simulink model "mpc_model_dual_module_currentcontroller"  (R2019a)
settings: Solver=FixedStepAuto  StartTime=0.0  StopTime=Tfinal  RelTol=1e-3
values from neighbouring files (symbols this model uses):
  A = [-0.0285 -0.0014; -0.0371 -0.1476]    [model.m]
  DCLINK_Cap = 1000e-12    (= 1e-09)    [mpc_model_parameters.m]    (also in mpc_model_parameters_dual_module.m = 0.001)
  FluxPM = MeanInducedVoltagePeak/(2*pi*100)    [mpc_model_parameters.m]    (also in mpc_model_parameters_dual_module.m)
  Inertia = 1e-2    (= 0.01)    [mpc_model_parameters.m]    (also in mpc_model_parameters_dual_module.m)
  iqrated = Trated/(1.5*PolePairs*FluxPM)    [mpc_model_parameters.m]    (also in mpc_model_parameters_dual_module.m)
  Ki = 8    [mpc_model_parameters_dual_module.m]
  Kp = 0.8    [mpc_model_parameters_dual_module.m]
  Ls = 3.5e-3    (= 0.0035)    [MPC_id_iq.m]    (also in mpc_model_parameters.m = 0.00351; mpc_model_parameters_dual_module.m = 0.00343)
  M1_FaultTime = 0.25    [mpc_model_parameters_dual_module.m]
  M2_FaultTime = 20    [mpc_model_parameters_dual_module.m]
  MeanLd = (1/12)*(Module1Phase_A_Ld+Module1Phase_B_Ld+Module1Phase_C_Ld+     Module2Phase_A_Ld+Module2Phase_B_Ld+Module2Phase_C_Ld+     Module3Phase_A_Ld+Module3Phase_B_Ld+Module3Phase_C_Ld+     Module4Phase_A_Ld+Module4Phase_B_Ld+Module4Phase_C_Ld)    [mpc_model_parameters.m]    (also in mpc_model_parameters_dual_module.m)
  MeanLq = (1/12)*(Module1Phase_A_Lq+Module1Phase_B_Lq+Module1Phase_C_Lq+     Module2Phase_A_Lq+Module2Phase_B_Lq+Module2Phase_C_Lq+     Module3Phase_A_Lq+Module3Phase_B_Lq+Module3Phase_C_Lq+     Module4Phase_A_Lq+Module4Phase_B_Lq+Module4Phase_C_Lq)    [mpc_model_parameters.m]    (also in mpc_model_parameters_dual_module.m)
  PI_Frequency = 5000    [mpc_model_parameters_dual_module.m]
  PI_Sat = iqrated*2    [mpc_model_parameters_dual_module.m]
  PI_Ts = 1/PI_Frequency    (= 0.0002)    [mpc_model_parameters_dual_module.m]
  PolePairs = 10    [mpc_model_parameters.m]    (also in mpc_model_parameters_dual_module.m)
  RefModeSelection = 1    [mpc_model_parameters_dual_module.m]
  Rin = 1e-3    (= 0.001)    [mpc_model_parameters.m]    (also in mpc_model_parameters_dual_module.m)
  Rs = 0.531    [Loss_Distribution.m]    (also in MPC_id_iq.m; mpc_model_parameters.m = 0.321; mpc_model_parameters_dual_module.m = 0.539)
  Sampling_time = 1e-6    (= 1e-06)    [mpc_model_parameters.m]    (also in mpc_model_parameters_dual_module.m)
  SpeedRef1 = 50    [mpc_model_parameters.m]    (also in mpc_model_parameters_dual_module.m = 35)
  SpeedRef2 = 100    [mpc_model_parameters.m]    (also in mpc_model_parameters_dual_module.m = 35)
  SpeedRefUpdateTime = 0.25    [mpc_model_parameters.m]    (also in mpc_model_parameters_dual_module.m = 1.75)
  Tload1 = 5    [mpc_model_parameters.m]    (also in mpc_model_parameters_dual_module.m = 30)
  Tload2 = 10    [mpc_model_parameters.m]    (also in mpc_model_parameters_dual_module.m = 63.6619772368)
  TloadUpdateTime = 0.5    [mpc_model_parameters.m]    (also in mpc_model_parameters_dual_module.m)
  Vdc = 50    [mpc_model_parameters.m]    (also in mpc_model_parameters_dual_module.m = 40)
  Vin = Vdc + Rin*(Pout/Vdc)    (= 50.04)    [mpc_model_parameters.m]    (also in mpc_model_parameters_dual_module.m = 40.05)
  ViscousFriction = 1e-3    (= 0.001)    [mpc_model_parameters.m]    (also in mpc_model_parameters_dual_module.m)
undefined symbols (not defined in the file or in its folder): DiscIntNeverNeededParam, LoadResistance, VoltageConstant_omega
libraries: dspsigops x30, powerlib x27, dspswit3 x19, powerlib_meascontrol x11, fl_lib x5, simulink x4, nesl_utility x3, sdl_lib x1
(part 1 of 3)
settings Model: Creator=hakan  LastModifiedBy=hakan
settings SolverCC: ZeroCrossAlgorithm=Adaptive
settings DebuggingCC: IgnoredZcDiagnostic=none  UnconnectedInputMsg=none  UnconnectedOutputMsg=none  UnconnectedLineMsg=none

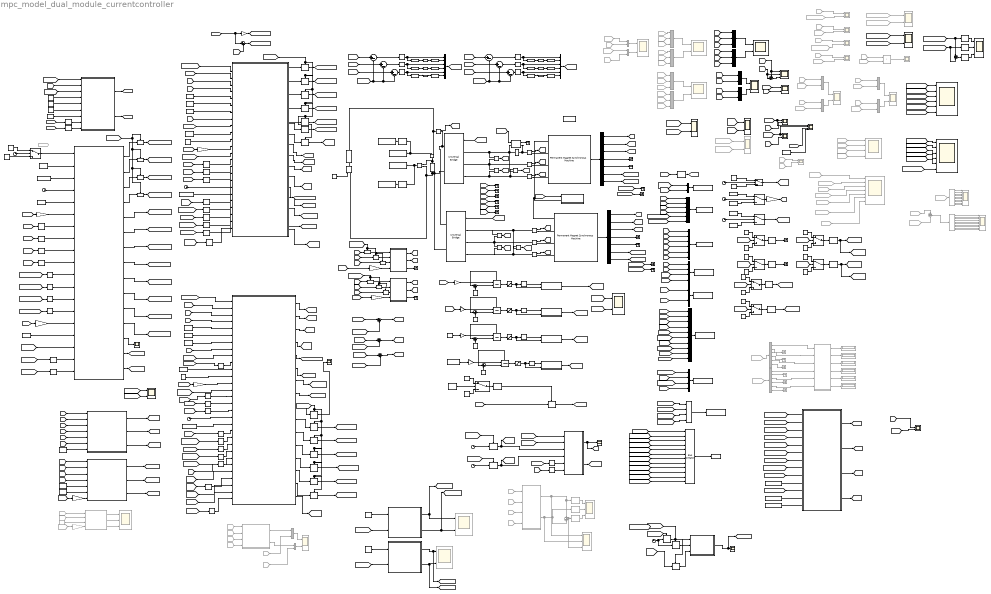
== system mpc_model_dual_module_currentcontroller ==
  note: M1_thetam & M2_thetam will be the but they are seperated anyway
  A_DCLINK_current : ToWorkspace  VariableName=M1_DCLINK_current  SaveFormat=Structure With Time  SampleTime=-1
  A_DCLINK_current_rms : ToWorkspace  VariableName=M1_DCLINK_current_rms  SaveFormat=Structure With Time  SampleTime=-1
  A_DCLINK_voltage : ToWorkspace  VariableName=M1_DCLINK_voltage  SaveFormat=Structure With Time  SampleTime=-1
  A_DCLINK_voltage_mean : ToWorkspace  VariableName=M1_DCLINK_voltage_mean  SaveFormat=Structure With Time  SampleTime=-1
  Bus Creator : BusCreator  Inputs=6
  Bus Creator1 : BusCreator  Inputs=6
  Bus Creator{3,10..12} (4 alike) : BusCreator  Inputs=2
  Bus Creator{13..14,17..20} (6 alike) : BusCreator  Commented=on  Inputs=2
  Bus Creator15 : BusCreator  Inputs=10
  Bus Creator16 : BusCreator  Inputs=4
  Bus Creator2 : BusCreator  Inputs=4
  Bus Creator21 : BusCreator  Inputs=4
  Bus Creator22 : BusCreator  Inputs=12
  Bus Creator{4..7} (4 alike) : BusCreator  Commented=on  Inputs=3
  Bus Creator8 : BusCreator  Inputs=3
  Bus Creator9 : BusCreator  Inputs=3
  Bus Selector : BusSelector  OutputSignals=Electromagnetic torque Te (N*m),Rotor speed wm (rad/s),Rotor angle thetam (rad),Stator current is_q (A),Stator current is_d (A),Stator voltage Vs_q (V),Stator voltage Vs_d (V)
  Bus Selector1 : BusSelector  OutputSignals=Electromagnetic torque Te (N*m),Rotor speed wm (rad/s),Rotor angle thetam (rad),Stator current is_q (A),Stator current is_d (A),Stator voltage Vs_q (V),Stator voltage Vs_d (V)
  Clock{,1..9} (10 alike) : Clock
  Compare To Zero{,1..3} (4 alike) : simulink/Logic and Bit Operations/Compare To Zero  relop===  OutDataTypeStr=boolean
  Constant : Constant  Value=Vin
  Constant{1..2,18,32} (4 alike) : Constant  Value=Rs
  Constant10 : Constant  Value=SpeedRef1
  Constant11 : Constant  Value=SpeedRef2
  Constant12 : Constant  Value=Tload2
  Constant13 : Constant  Value=M2_FaultTime
  Constant{5,14,26,31} (4 alike) : Constant  Value=Ls
  Constant{15,17,22,29,36,38..39,43,50,52} (10 alike) : Constant  Value=0
  Constant{16,23,27,30,37,44,49,51} (8 alike) : Constant
  Constant19 : Constant  Value=PolePairs
  Constant{4,6,20,34} (4 alike) : Constant  Value=FluxPM
  Constant21 : Constant  Value=Vdc
  Constant{7,24..25,41} (4 alike) : Constant  Value=1.02
  Constant28 : Constant  Value=M1_FaultTime
  Constant3 : Constant  Value=M1_FaultTime
  Constant33 : Constant  Value=PolePairs
  Constant35 : Constant  Value=Vdc
  Constant40 : Constant  Value=RefModeSelection
  Constant42 : Constant  Value=PI_Frequency
  Constant45 : Constant  Value=Ki
  Constant46 : Constant  Value=Kp
  Constant47 : Constant  Value=PI_Ts
  Constant48 : Constant  Value=PI_Sat
  Constant53 : Constant  Commented=on  Value=0
  Constant54 : Constant  Value=2*iqrated
  Constant55 : Constant  Value=5
  Constant56 : Constant  Value=15
  Constant8 : Constant  Value=Tload1
  Constant9 : Constant  Value=2000
  Controlled Voltage Source : powerlib/Electrical Sources/Controlled Voltage Source  Initialize=on  Source_Type=DC  Amplitude=0  Phase=0  Frequency=0  Measurements=None
      settings: SourceProductName=Simscape Electrical
  Current Measurement{,1..7} (8 alike) : powerlib/Measurements/Current Measurement  PhasorSimulation=off  OutputType=Complex  PSBequivalent=0
      settings: SourceProductName=Simscape Electrical
  DCLINK_Cap : powerlib/Elements/Series RLC Branch  LConnTagsString=__new0  RConnTagsString=__new0  BranchType=C  Resistance=1  Inductance=1e-3  SetiL0=off  InitialCurrent=0  Capacitance=DCLINK_Cap  Setx0=on  InitialVoltage=Vin  Measurements=None
      settings: SourceProductName=Simscape Electrical
  Data Type Conversion{1,3,5,12,14,16} (6 alike) : DataTypeConversion  OutDataTypeStr=boolean
  Data Type Conversion{2,4,6,13,15,17} (6 alike) : DataTypeConversion  OutDataTypeStr=double
  Delay{,1..21,23..29,32..33} (31 alike) : Delay  DelayLength=1
  Delay22 : Delay  DelayLength=1  InitialCondition=1
  Delay30 : Delay  DelayLength=1  InitialCondition=1
  Delay31 : Delay
  Demux : Demux  Commented=on  Outputs=10
  Demux1 : Demux  Commented=on  Outputs=10
  Demux2 : Demux  Commented=on  Outputs=6
  Demux3 : Demux  Commented=on  Outputs=6
  Discrete-Time Integrator{1..4} (4 alike) : DiscreteIntegrator  ExternalReset=falling  SampleTime=Sampling_time  UpperSaturationLimit=1  LowerSaturationLimit=0  ShowStatePort=on  ICPrevOutput=DiscIntNeverNeededParam  ICPrevScaledInput=DiscIntNeverNeededParam
  Display{1..6} (6 alike) : Display  Commented=on
  Edge Detector{1,3,5..9} (7 alike) : dspswit3/Edge Detector  InputProcessing=Columns as channels (frame based)
      settings: SourceProductName=DSP System Toolbox  SourceProductBaseCode=DS
  Error : Scope  Commented=on  NumInputPorts=10
  From10 : From  Commented=on  GotoTag=M1_Vbc
  From11 : From  Commented=on  GotoTag=M1_Vca
  From112 : From  Commented=on  GotoTag=PI_output
  From122 : From  Commented=on  GotoTag=M2_thetam
  From{126,172,246,250,262} (5 alike) : From  Commented=on  GotoTag=M2_ids
  From{49,127,171,244,248,260} (6 alike) : From  Commented=on  GotoTag=M1_ids
  From131 : From  Commented=on  GotoTag=M1_idref
  From137 : From  Commented=on  GotoTag=M1_cond_loss
  From138 : From  Commented=on  GotoTag=M1_core_loss
  From139 : From  Commented=on  GotoTag=M2_core_loss
  From140 : From  Commented=on  GotoTag=M2_cond_loss
  From141 : From  Commented=on  GotoTag=Total_cond_loss
  From142 : From  Commented=on  GotoTag=Total_core_loss
  From{143,166,242,311} (4 alike) : From  Commented=on  GotoTag=M1_iqref
  From144 : From  Commented=on  GotoTag=M2_iqref
  From{94,146,245,249,261} (5 alike) : From  Commented=on  GotoTag=M1_iqs
  From{148,247,251,263} (4 alike) : From  Commented=on  GotoTag=M2_iqs
  From156 : From  Commented=on  GotoTag=Total_loss
  From158 : From  Commented=on  GotoTag=Total_loss
  From159 : From  Commented=on  GotoTag=M2_loss
  From160 : From  Commented=on  GotoTag=M1_loss
  From161 : From  Commented=on  GotoTag=Mean_loss
  From164 : From  Commented=on  GotoTag=M1_opt
  From165 : From  Commented=on  GotoTag=M2_opt
  From167 : From  Commented=on  GotoTag=M2_iqref
  From170 : From  Commented=on  GotoTag=M2_idref
  From20 : From  Commented=on  GotoTag=M2_IqRipplePrediction
  From234 : From  Commented=on  GotoTag=M1_magneticloss
  From235 : From  Commented=on  GotoTag=M2_magneticloss
  From238 : From  Commented=on  GotoTag=M1_wmech
  From239 : From  Commented=on  GotoTag=M1_Te
  From240 : From  Commented=on  GotoTag=M2_idref
  From241 : From  Commented=on  GotoTag=M2_iqref
  From243 : From  Commented=on  GotoTag=M1_idref
  From252 : From  Commented=on  GotoTag=M1_Te
  From253 : From  Commented=on  GotoTag=M2_Te
  From309 : From  Commented=on  GotoTag=iq_2_store
  From310 : From  Commented=on  GotoTag=iq_2_store
  From32 : From  Commented=on  GotoTag=M1_va_1
  From33 : From  Commented=on  GotoTag=M1_vb_1
  From34 : From  Commented=on  GotoTag=M1_vc_1
  From42 : From  Commented=on  GotoTag=M1_mpcgate
  From58 : From  Commented=on  GotoTag=M2_Vbc
  From59 : From  Commented=on  GotoTag=M2_Vca
  From6 : From  Commented=on  GotoTag=M1_mpcgate
  From60 : From  Commented=on  GotoTag=M2_Vab
  From61 : From  Commented=on  GotoTag=M2_va_1
  From62 : From  Commented=on  GotoTag=M2_vb_1
  From63 : From  Commented=on  GotoTag=M2_vc_1
  From76 : From  Commented=on  GotoTag=M1_IqRipplePrediction
  From9 : From  Commented=on  GotoTag=M1_Vab
  Gain1 : Gain  Gain=2*pi/60
  Gain11 : Gain  Gain=0.5
  Gain{7..8,12,14} (4 alike) : Gain  Gain=2
  Gain{3..6,9,13,15} (7 alike) : Gain  Gain=PolePairs
  Gain2 : Gain  Commented=on  Gain=PolePairs
  Ideal Switch : powerlib/Power Electronics/Ideal Switch  Ron=0.001  Lon=0  IC=0  Rs=1e5  Cs=inf  Measurements=on
      settings: SourceProductName=Simscape Electrical
  Inverter1 : powerlib/Power Electronics/Universal Bridge  Arms=3  SnubberResistance=1e5  SnubberCapacitance=inf  Device=IGBT / Diodes  Ron=0.65e-3  Lon=0  ForwardVoltages="[  0  0  ]"  ForwardVoltage=0  GTOparameters=[ 10e-6 , 20e-6 ]  IGBTparameters=[ 1e-6 , 2e-6 ]  Measurements=All voltages and currents  Measurements_2=None  converterType=Rectifier
      settings: SourceProductName=Simscape Electrical
  Inverter2 : powerlib/Power Electronics/Universal Bridge  Arms=3  SnubberResistance=1e5  SnubberCapacitance=inf  Device=IGBT / Diodes  Ron=0.65e-3  Lon=0  ForwardVoltages="[  0  0  ]"  ForwardVoltage=0  GTOparameters=[ 10e-6 , 20e-6 ]  IGBTparameters=[ 1e-6 , 2e-6 ]  Measurements=All voltages and currents  Measurements_2=None  converterType=Rectifier
      settings: SourceProductName=Simscape Electrical
  Logical Operator{1..3,6..8} (6 alike) : Logic  Operator=NOT  AllPortsSameDT=off  OutDataTypeStr=boolean
  M1 Prediction : MATLAB Function  TreatAsAtomicUnit=on
  M2 Prediction : MATLAB Function  TreatAsAtomicUnit=on
  MATLAB Function : MATLAB Function  Commented=on  TreatAsAtomicUnit=on
  MATLAB Function1 : MATLAB Function  TreatAsAtomicUnit=on
  MATLAB Function10 : MATLAB Function  TreatAsAtomicUnit=on
  MATLAB Function11 : MATLAB Function  Commented=on  TreatAsAtomicUnit=on
  MATLAB Function12 : MATLAB Function  Commented=on  TreatAsAtomicUnit=on
  MATLAB Function13 : MATLAB Function  TreatAsAtomicUnit=on
  MATLAB Function14 : MATLAB Function  TreatAsAtomicUnit=on
  MATLAB Function15 : MATLAB Function  TreatAsAtomicUnit=on
  MATLAB Function2 : MATLAB Function  TreatAsAtomicUnit=on
  MATLAB Function3 : MATLAB Function  TreatAsAtomicUnit=on
  MATLAB Function4 : MATLAB Function  TreatAsAtomicUnit=on
  MATLAB Function5 : MATLAB Function  TreatAsAtomicUnit=on
  MATLAB Function6 : MATLAB Function  TreatAsAtomicUnit=on
  MATLAB Function7 : MATLAB Function  TreatAsAtomicUnit=on
  MATLAB Function8 : MATLAB Function  TreatAsAtomicUnit=on
  MATLAB Function9 : MATLAB Function  TreatAsAtomicUnit=on
  Mean : powerlib_meascontrol/Measurements/Mean  Freq=THD_mean_frequency  Vinit=0  Ts=Sampling_time
      settings: SourceProductName=Simscape Electrical
  Mean Switching Frequency : Subsystem  Commented=on
  Mean1 : powerlib_meascontrol/Measurements/Mean  Freq=1/0.2  Vinit=0  Ts=0
      settings: SourceProductName=Simscape Electrical
  Mean2 : powerlib_meascontrol/Measurements/Mean  Freq=5  Vinit=0  Ts=Sampling_time
      settings: SourceProductName=Simscape Electrical
  Mean3 : powerlib_meascontrol/Measurements/Mean  Freq=1/0.2  Vinit=0  Ts=0
      settings: SourceProductName=Simscape Electrical
  Mean4 : powerlib_meascontrol/Measurements/Mean  Freq=1/0.2  Vinit=0  Ts=0
      settings: SourceProductName=Simscape Electrical
  Mean5 : powerlib_meascontrol/Measurements/Mean  Commented=on  Freq=1/0.2  Vinit=0  Ts=0
      settings: SourceProductName=Simscape Electrical
  Mean6 : powerlib_meascontrol/Measurements/Mean  Commented=on  Freq=1/0.2  Vinit=0  Ts=0
      settings: SourceProductName=Simscape Electrical
  Mean7 : powerlib_meascontrol/Measurements/Mean  Commented=on  Freq=1/0.2  Vinit=0  Ts=0
      settings: SourceProductName=Simscape Electrical
  Mechanical Subsystem : Subsystem
  Multimeter : powerlib/Measurements/Multimeter  PhasorSimulation=off  OutputType=Complex  sel=27  L=32  Gain=1  yselected={'Isw1: Inverter1'};  PSBOutputType=1  PSBequivalent=0  AxesSetting=[0,0.1,-100,100]  Display=0  SavedBlockNames=-11
      settings: SourceProductName=Simscape Electrical
  Multimeter1 : powerlib/Measurements/Multimeter  PhasorSimulation=off  OutputType=Complex  sel=21  L=32  Gain=1  yselected={'Isw1: Inverter2'};  PSBOutputType=1  PSBequivalent=0  AxesSetting=[0,0.1,-100,100]  Display=0  SavedBlockNames=-11
      settings: SourceProductName=Simscape Electrical
  Mux : Mux  Commented=on  Inputs=2
  Mux1 : Mux  Inputs=6
  Mux2 : Mux  Commented=on  Inputs=2
  Mux4 : Mux  Inputs=6
  Permanent Magnet Synchronous Machine : powerlib/Machines/Permanent Magnet Synchronous Machine  NbPhases=3  FluxDistribution=Sinusoidal  RotorType=Round  MechanicalLoad=Mechanical rotational port  PresetModel=No  ShowDetailedParameters=on  MeasurementBus=off  Resistance=Rs  Inductance=8.5e-3  dqInductances=[MeanLd,MeanLq]  La=Ls  MachineConstant=Flux linkage established by magnets (V.s)  Flux=0.18074  VoltageCst=327.8261  TorqueCst=2.7111  Flat=120  Mechanical=[Inertia ViscousFriction PolePairs 0]  PolePairs=4  InitialConditions=[0,0, 0,0]  InitialConditions5ph=[0 0 0 0 0 0]  TsPowergui=0  TsBlock=-1  RefAngle=90 degrees behind phase A axis (modified Park)
  Permanent Magnet Synchronous Machine1 : powerlib/Machines/Permanent Magnet Synchronous Machine  NbPhases=3  FluxDistribution=Sinusoidal  RotorType=Round  MechanicalLoad=Mechanical rotational port  PresetModel=No  ShowDetailedParameters=on  MeasurementBus=off  Resistance=Rs  Inductance=8.5e-3  dqInductances=[MeanLd,MeanLq]  La=Ls  MachineConstant=Flux linkage established by magnets (V.s)  Flux=0.18074  VoltageCst=327.8261  TorqueCst=2.7111  Flat=120  Mechanical=[Inertia ViscousFriction PolePairs 0]  PolePairs=4  InitialConditions=[0,0, 0,0]  InitialConditions5ph=[0 0 0 0 0 0]  TsPowergui=0  TsBlock=-1  RefAngle=90 degrees behind phase A axis (modified Park)
  Product : Product  Commented=on
  RMS1 : powerlib_meascontrol/Measurements/RMS  TrueRMS=on  Freq=Load_Nominal_Freq  RMSInit=10  Ts=Sampling_time
      settings: SourceProductName=Simscape Electrical
  Relay{,1..5} (6 alike) : Relay
  Rin : powerlib/Elements/Series RLC Branch  LConnTagsString=__new0  RConnTagsString=__new0  BranchType=R  Resistance=Rin  Inductance=1e-3  SetiL0=off  InitialCurrent=0  Capacitance=1000e-6  Setx0=off  InitialVoltage=0  Measurements=None
      settings: SourceProductName=Simscape Electrical
  Sample and Hold{,1..29} (30 alike) : dspsigops/Sample and Hold  trig=Rising edge  initCond=0  latchinput=off
  Saturation{1..3,12} (4 alike) : Saturate  UpperLimit=1  LowerLimit=0
  Sawtooth Generator : powerlib_meascontrol/Pulse & Signal Generators/Sawtooth Generator  Freq=1000  Phase=180  Ts=0
      settings: SourceProductName=Simscape Electrical
  Scope : Scope  NumInputPorts=3
  Scope{1,5..6,8..10,12..13,22,30,35} (11 alike) : Scope  NumInputPorts=2
  Scope{2,4,7,11,17..19,21,24..28,37..38} (15 alike) : Scope  Commented=on  NumInputPorts=2
  Scope14 : Scope  Commented=on  NumInputPorts=3
  Scope{15,29,34,39} (4 alike) : Scope
  Scope16 : Scope  Commented=on  NumInputPorts=4
  Scope20 : Scope  NumInputPorts=4
  Scope23 : Scope  Commented=on
  Scope3 : Scope  Commented=on  NumInputPorts=7
  Scope31 : Scope  NumInputPorts=3
  Scope32 : Scope  Commented=on  NumInputPorts=3
  Scope33 : Scope  Commented=on  NumInputPorts=3
  Scope36 : Scope  NumInputPorts=6
  Scope40 : Scope  NumInputPorts=6
  Scope42 : Scope  Commented=on  NumInputPorts=10
  Series RLC Branch : powerlib/Elements/Series RLC Branch  LConnTagsString=__new0  RConnTagsString=__new0  BranchType=R  Resistance=5000  Inductance=1e-3  SetiL0=off  InitialCurrent=0  Capacitance=1e-6  Setx0=off  InitialVoltage=0  Measurements=None
      settings: SourceProductName=Simscape Electrical
  Sum : Sum  Inputs=|++
  Sum1 : Sum  Inputs=++|
  Sum{10..12,15} (4 alike) : Sum  Inputs=|-+
  Sum{2,4..6,8..9,13} (7 alike) : Sum  Inputs=|+-
  Sum14 : Sum
  Sum16 : Sum  Commented=on
  Sum18 : Sum  Commented=on  Inputs=+-
  Sum3 : Sum  Inputs=|++
  Sum7 : Sum  Inputs=|++
  Switch : Switch  Criteria=u2 > Threshold  Threshold=SpeedRefUpdateTime
  Switch1 : Switch  Criteria=u2 > Threshold  Threshold=TloadUpdateTime
  Switch11 : Switch  Criteria=u2 > Threshold  Threshold=0.25
  Switch2 : Switch  Criteria=u2 ~= 0
  Switch3 : Switch  Criteria=u2 > Threshold  Threshold=M1_FaultTime
  Switch4 : Switch  Criteria=u2 ~= 0
  Switch5 : Switch  Threshold=0.99
  Switch6 : Switch  Criteria=u2 ~= 0
  Switch7 : Switch  Threshold=(rand/2+1.5)/2
  Switch8 : Switch  Threshold=1
  Switch9 : Switch  Threshold=1
  Terminator{,2..9,15..24} (19 alike) : Terminator
  Terminator{1,10..14} (6 alike) : Terminator  Commented=on
  To Workspace : ToWorkspace  VariableName=FswPhases  SaveFormat=Timeseries  SampleTime=-1
  To Workspace1 : ToWorkspace  VariableName=Simout_PhaseCurrents_abc  SaveFormat=Timeseries  SampleTime=-1
  To Workspace2 : ToWorkspace  VariableName=Simout_PhaseCurrents_dq  SaveFormat=Timeseries  SampleTime=-1
  To Workspace3 : ToWorkspace  VariableName=Simout_TorqueSpeedMeas  SaveFormat=Timeseries  SampleTime=-1
  To Workspace4 : ToWorkspace  VariableName=Simout_TorqueSpeedRef  SaveFormat=Timeseries  SampleTime=-1
  To Workspace5 : ToWorkspace  VariableName=Simout_Fsw  SaveFormat=Timeseries  SampleTime=-1
  To Workspace6 : ToWorkspace  VariableName=Simout_losses  SaveFormat=Timeseries  SampleTime=-1
  To Workspace7 : ToWorkspace  VariableName=Simout_Reference_Idq  SaveFormat=Timeseries  SampleTime=-1
  To Workspace8 : ToWorkspace  VariableName=InverterLoss  SaveFormat=Timeseries  SampleTime=-1
  Voltage Measurement{,1..6} (7 alike) : powerlib/Measurements/Voltage Measurement  PhasorSimulation=off  OutputType=Complex  PSBequivalent=0
      settings: SourceProductName=Simscape Electrical
  module 1 abc to dq1 : MATLAB Function  TreatAsAtomicUnit=on
  module 2 abc to dq1 : MATLAB Function  TreatAsAtomicUnit=on
  powergui : powerlib/powergui  Priority=1  SimulationMode=Discrete  SampleTime=Sampling_time  frequency=60  Iterations=50  frequencyindice=0  Pbase=100e6  ErrMax=1e-4  UnitsV=kV  UnitsW=MW  buscounter=0  FunctionMessages=off  echomessages=off  EnableUseOfTLC=off  CurrentSourceSwitches=off  DisableSnubberDevices=off  DisableRonSwitches=off  DisableVfSwitches=off  DisplayEquations=off  AutomaticDiscreteSolvers=off  SolverType=Tustin/Backward Euler (TBE)  Interpol=off  ExternalGateDelay=off  methode=off  Ts=100  x0status=blocks  SPID=on  SwTol=0  HookPort=off  NonlinearTolerance=0  nMaxIteration=15  ContinueOnMaxIteration=off  RestoreLinks=warning  ResistiveCurrentMeasurement=off  Frange=[0:2:500]  Ylog=off  Xlog=on  ShowGrid=off  save=off  variable=ZData  structure=0  ZoomFFT=off  StartTime=0.0  cycles=1  DisplayStyle=1  fundamental=60  FreqAxis=off  MaxFrequency=1000  frequencyindicesteady=1  RmsSteady=1  display=off
      settings: SourceProductName=Simscape Electrical
  wires:
  Voltage Measurement3/1 -> Mean/1, A_DCLINK_voltage/1
  RMS1/1 -> A_DCLINK_current_rms/1
  Constant/1 -> Controlled Voltage Source/1
  Mean/1 -> A_DCLINK_voltage_mean/1
  Current Measurement/1 -> RMS1/1, A_DCLINK_current/1
  Permanent Magnet Synchronous Machine/1 -> Bus Selector/1
  Bus Selector/1 -> [M1_Te]  "<Electromagnetic torque Te (N*m)>"
  Bus Selector/2 -> [M1_wmech]  "<Rotor speed wm (rad/s)>"
  Current Measurement1/1 -> [M1_Ia]
  Current Measurement2/1 -> [M1_Ib]
  Current Measurement3/1 -> [M1_Ic]
  Bus Selector/3 -> [M1_thetam]  "<Rotor angle thetam (rad)>"
  Bus Selector/4 -> Terminator4/1  "<Stator current is_q (A)>"
  Bus Selector/5 -> Terminator5/1  "<Stator current is_d (A)>"
  Voltage Measurement/1 -> [M1_Vab]
  Voltage Measurement1/1 -> [M1_Vbc]
  Voltage Measurement2/1 -> [M1_Vca]
  Bus Selector/6 -> [M1_vsq_actual]  "<Stator voltage Vs_q (V)>"
  Bus Selector/7 -> [M1_vsd_actual]  "<Stator voltage Vs_d (V)>"
  [M1_mpcgate] -> Inverter1/1
  [M1_iqs] -> Bus Creator1/2  "M1_iqs"
  [M1_ids] -> Bus Creator1/1  "M1_ids"
  Constant10/1 -> Switch/3
  Constant11/1 -> Switch/1
  Switch/1 -> Gain1/1
  Clock/1 -> Switch/2
  Clock1/1 -> Switch1/2
  Constant12/1 -> Switch1/1
  Constant8/1 -> Switch1/3
  Switch1/1 -> [Combined_Tload]
  Bus Creator/1 -> To Workspace1/1  "Iabc"
  Bus Creator1/1 -> To Workspace2/1  "Idq"
  Bus Creator2/1 -> To Workspace3/1
  Gain1/1 -> [wref]
  [Combined_Tload] -> Bus Creator3/1  "Combined_Tload"
  [wref] -> Bus Creator3/2  "wref"
  Bus Creator3/1 -> To Workspace4/1
  [M1_Ib] -> Bus Creator/2  "M1_Ib"
  [M1_Ia] -> Bus Creator/1  "M1_Ia"
  [M1_Ic] -> Bus Creator/3  "M1_Ic"
  [M1_iqs] -> Bus Creator10/1  "M1_iqs"
  [M1_ids] -> Bus Creator10/2  "M1_ids"
  [M1_Te] -> Bus Creator2/1  "M1_Te"
  [M1_Te] -> Sum1/1, Scope/1  "M1_Te"
  [M1_wmech] -> Scope1/1  "M1_wmech"
  [M1_FaultTrig] -> Ideal Switch/1
  Constant16/1 -> Switch3/3
  Clock2/1 -> Switch3/2
  Constant15/1 -> Switch3/1
  Switch3/1 -> [M1_FaultTrig]
  [M1_wmech] -> Bus Creator2/3  "M1_wmech"
  [M2_Te] -> Bus Creator2/2  "M2_Te"
  Bus Selector1/7 -> [M2_vsd_actual]  "<Stator voltage Vs_d (V)>"
  Bus Selector1/6 -> [M2_vsq_actual]  "<Stator voltage Vs_q (V)>"
  Bus Selector1/5 -> Terminator7/1  "<Stator current is_d (A)>"
  Bus Selector1/4 -> Terminator6/1  "<Stator current is_q (A)>"
  Bus Selector1/3 -> [M2_thetam]  "<Rotor angle thetam (rad)>"
  Bus Selector1/2 -> [M2_wmech]  "<Rotor speed wm (rad/s)>"
  Bus Selector1/1 -> [M2_Te]  "<Electromagnetic torque Te (N*m)>"
  Permanent Magnet Synchronous Machine1/1 -> Bus Selector1/1
  Current Measurement4/1 -> [M2_Ia]
  Current Measurement5/1 -> [M2_Ib]
  Current Measurement6/1 -> [M2_Ic]
  Voltage Measurement5/1 -> [M2_Vbc]
  Voltage Measurement4/1 -> [M2_Vab]
  Voltage Measurement6/1 -> [M2_Vca]
  [M2_wmech] -> Bus Creator2/4  "M2_wmech"
  [M2_ids] -> Bus Creator1/3  "M2_ids"
  [M2_iqs] -> Bus Creator1/4  "M2_iqs"
  [M2_Ic] -> Bus Creator/6  "M2_Ic"
  [M2_Ia] -> Bus Creator/4  "M2_Ia"
  [M2_Ib] -> Bus Creator/5  "M2_Ib"
  [M2_Te] -> Sum1/2, Scope/2  "M2_Te"
  From10/1 -> Bus Creator5/2
  From9/1 -> Bus Creator5/1
  From11/1 -> Bus Creator5/3
  From59/1 -> Bus Creator4/3
  From60/1 -> Bus Creator4/1
  From58/1 -> Bus Creator4/2
  Bus Creator4/1 -> Scope2/2  "M2_Vlinetoline_abc"
  Bus Creator5/1 -> Scope2/1  "M1_Vlinetoline_abc"
  Bus Creator7/1 -> Scope4/1  "M1_gate"
  Bus Creator6/1 -> Scope4/2  "M2_gate"
  From62/1 -> Bus Creator6/2
  From61/1 -> Bus Creator6/1
  From63/1 -> Bus Creator6/3
  From34/1 -> Bus Creator7/3
  From33/1 -> Bus Creator7/2
  From32/1 -> Bus Creator7/1
  Bus Creator9/1 -> Scope5/1  "M1_Iabc"
  Bus Creator8/1 -> Scope5/2  "M2_Iabc"
  [M2_Ib] -> Bus Creator8/2
  [M2_Ia] -> Bus Creator8/1
  [M2_Ic] -> Bus Creator8/3
  [M1_Ic] -> Bus Creator9/3
  [M1_Ia] -> Bus Creator9/1
  [M1_Ib] -> Bus Creator9/2
  Bus Creator10/1 -> Scope8/1  "M1_iqds"
  [M2_ids] -> Bus Creator11/2  "M2_ids"
  [M2_iqs] -> Bus Creator11/1  "M2_iqs"
  Bus Creator11/1 -> Scope8/2  "M2_iqds"
  [M2_mpcgate] -> Inverter2/1
  Sum1/1 -> Scope/3
  Relay/1 -> Mux4/1, Data Type Conversion14/1
  Mux4/1 -> [M1_mpcgate]
  Sum5/1 -> Relay1/1
  Logical Operator8/1 -> Data Type Conversion13/1
  Logical Operator7/1 -> Data Type Conversion17/1
  [M1_DutyB] -> Sum5/1
  Sum2/1 -> Relay/1
  Data Type Conversion15/1 -> Mux4/2
  Sum6/1 -> Relay2/1
  Logical Operator6/1 -> Data Type Conversion15/1
  Data Type Conversion12/1 -> Logical Operator8/1
  Relay1/1 -> Data Type Conversion16/1, Mux4/3
  Data Type Conversion13/1 -> Mux4/6
  [M1_CarrierSignal] -> Sum2/2, Sum5/2, Sum6/2
  Data Type Conversion14/1 -> Logical Operator6/1
  [M1_DutyC] -> Sum6/1
  Relay2/1 -> Data Type Conversion12/1, Mux4/5
  [M1_DutyA] -> Sum2/1
  Data Type Conversion16/1 -> Logical Operator7/1
  Data Type Conversion17/1 -> Mux4/4
  Constant29/1 -> Switch4/1
  Constant30/1 -> Switch4/3
  [M1_CarrierSignal] -> Switch4/2
  Data Type Conversion6/1 -> Mux1/4
  Data Type Conversion5/1 -> Logical Operator2/1
  [M2_DutyA] -> Sum4/1
  Relay5/1 -> Mux1/5, Data Type Conversion1/1
  [M2_DutyC] -> Sum9/1
  Data Type Conversion3/1 -> Logical Operator1/1
  [M2_CarrierSignal] -> Sum9/2, Sum8/2, Sum4/2
  Data Type Conversion2/1 -> Mux1/6
  Relay4/1 -> Mux1/3, Data Type Conversion5/1
  Data Type Conversion1/1 -> Logical Operator3/1
  Logical Operator1/1 -> Data Type Conversion4/1
  Sum9/1 -> Relay5/1
  Data Type Conversion4/1 -> Mux1/2
  Sum4/1 -> Relay3/1
  [M2_DutyB] -> Sum8/1
  Logical Operator2/1 -> Data Type Conversion6/1
  Logical Operator3/1 -> Data Type Conversion2/1
  Sum8/1 -> Relay4/1
  Mux1/1 -> [M2_mpcgate]
  Relay3/1 -> Data Type Conversion3/1, Mux1/1
  [M2_CarrierSignal] -> Switch2/2
  Constant23/1 -> Switch2/3
  Constant22/1 -> Switch2/1
  [M1_fsw_out] -> Scope6/1  "M1_fsw"
  [M2_fsw_out] -> Scope6/2  "M2_fsw"
  From76/1 -> Scope7/1  "M1_iqripple"
  From20/1 -> Scope7/2  "M2_iqripple"
  Discrete-Time Integrator2/1 -> Saturation1/1
  Sum10/1 -> Discrete-Time Integrator2/2
  Compare To Zero/1 -> MATLAB Function1/1(pulse)
  MATLAB Function1/1(outputwave) -> [M1_CarrierSignal]
  [M1_fsw_out] -> Gain8/1
  Saturation1/1 -> MATLAB Function1/2(inputwave), Compare To Zero/1
  Discrete-Time Integrator2/State -> Sum10/1
  Constant24/1 -> Sum10/2
  Constant25/1 -> Sum12/2
  Discrete-Time Integrator3/State -> Sum12/1
  Saturation2/1 -> Compare To Zero1/1, MATLAB Function2/2(inputwave)
  [M2_fsw_out] -> Gain7/1
  Compare To Zero1/1 -> MATLAB Function2/1(pulse)
  Sum12/1 -> Discrete-Time Integrator3/2
  Discrete-Time Integrator3/1 -> Saturation2/1
  Gain7/1 -> Discrete-Time Integrator3/1
  Gain8/1 -> Discrete-Time Integrator2/1
  Bus Creator12/1 -> To Workspace5/1
  [M2_fsw_out] -> Bus Creator12/2  "M2_fsw_out"
  [M1_fsw_out] -> Bus Creator12/1  "M1_fsw_out"
  [M1_IqRipplePrediction] -> Bus Creator1/5  "M1_iqripple"
  [M2_IqRipplePrediction] -> Bus Creator1/6  "M2_iqripple"
  [M2_iqref] -> Scope20/2, Scope10/1  "M2_iqref"
  [M2_iqs] -> Scope10/2  "M2_iqs"
  [M1_iqref] -> Scope20/1, Scope9/1  "M1_iqref"
  [M1_iqs] -> Scope9/2  "M1_iqs"
  [M1_ids] -> M1 Prediction/3(IdMeasured)
  [M1_DutyC] -> Delay15/1
  Delay7/1 -> M1 Prediction/20(IqRipplePrediction_prev)
  [M1_iqs] -> M1 Prediction/4(IqMeasured)
  M1 Prediction/8(DutyA) -> [M1_DutyA]
  Gain6/1 -> M1 Prediction/12(ElectricalAngle)
  [M1_DutyB] -> Delay10/1
  [M1_DutyA] -> Delay9/1
  [M1_idref] -> M1 Prediction/2(idref)
  M1 Prediction/12(IqRipplePrediction) -> [M1_IqRipplePrediction]
  Delay9/1 -> M1 Prediction/14(DutyA_prev)
  M1 Prediction/9(DutyB) -> [M1_DutyB]
  Constant31/1 -> M1 Prediction/5(Ls)
  Delay10/1 -> M1 Prediction/15(DutyB_prev)
  M1 Prediction/10(DutyC) -> [M1_DutyC]
  Constant28/1 -> M1 Prediction/18(FaultOccuranceTime)
  [M1_IqRipplePrediction] -> Delay7/1
  Delay8/1 -> M1 Prediction/19(FswSelected_prev)
  Delay15/1 -> M1 Prediction/16(DutyC_prev)
  Clock5/1 -> M1 Prediction/17(SimulationClock)
  [M1_switching_pulse] -> M1 Prediction/13(InterruptPulse)
  Constant33/1 -> M1 Prediction/7(PolePairs)
  [wmech_lowrate] -> M1 Prediction/9(ShaftAngularSpeed)
  [M1_thetam] -> Gain6/1
  Constant35/1 -> M1 Prediction/11(Vdc)
  Constant34/1 -> M1 Prediction/10(FluxPM)
  Constant32/1 -> M1 Prediction/6(Rs)
  [M1_fsw_out] -> Delay8/1
  M1 Prediction/11(FswSelected) -> [M1_fsw_out]
  M2 Prediction/4(FswSelected) -> [M2_fsw_out]
  [M2_fsw_out] -> Delay19/1
  Constant18/1 -> M2 Prediction/6(Rs)
  Constant20/1 -> M2 Prediction/11(FluxPM)
  Constant21/1 -> M2 Prediction/12(Vdc)
  [M2_thetam] -> Gain4/1
  [wmech_lowrate] -> M2 Prediction/9(ShaftAngularSpeed)
  Constant19/1 -> M2 Prediction/7(PolePairs)
  [M2_switching_pulse] -> M2 Prediction/14(InterruptPulse)
  Clock4/1 -> M2 Prediction/18(SimulationClock)
  Delay4/1 -> M2 Prediction/17(DutyC_prev)
  Delay19/1 -> M2 Prediction/20(FswSelected_prev)
  [M2_IqRipplePrediction] -> Delay18/1
  Constant13/1 -> M2 Prediction/19(FaultOccuranceTime)
  Delay3/1 -> M2 Prediction/16(DutyB_prev)
  Constant14/1 -> M2 Prediction/5(Ls)
  M2 Prediction/2(DutyB) -> [M2_DutyB]
  Delay20/1 -> M2 Prediction/15(DutyA_prev)
  M2 Prediction/5(IqRipplePrediction) -> [M2_IqRipplePrediction]
  [M2_DutyA] -> Delay20/1
  [M2_DutyB] -> Delay3/1
  [M2_iqref] -> M2 Prediction/1(iqref)
  Gain4/1 -> M2 Prediction/13(ElectricalAngle)
  M2 Prediction/1(DutyA) -> [M2_DutyA]
  [M2_iqs] -> M2 Prediction/4(IqMeasured)
  Delay18/1 -> M2 Prediction/21(IqRipplePrediction_prev)
  [M2_DutyC] -> Delay4/1
  [M2_ids] -> M2 Prediction/3(IdMeasured)
  [M1_iqref] -> M1 Prediction/1(iqref)
  From126/1 -> Scope11/2  "M2_ids"
  From127/1 -> Scope11/1  "M1_ids"
  [M2_idref] -> M2 Prediction/2(idref)
  MATLAB Function3/5(M1_iqref) -> [M1_Iq_opt_cost]
  MATLAB Function3/7(M2_iqref) -> [M2_Iq_opt_cost]
  Constant2/1 -> MATLAB Function3/2(Rs)
  MATLAB Function3/6(M1_idref) -> [M1_Id_opt_cost]
  MATLAB Function3/8(M2_idref) -> [M2_Id_opt_cost]
  Constant3/1 -> MATLAB Function3/3(M1_FaultTime)
  Clock3/1 -> MATLAB Function3/4(clock)
  [M1_thetam] -> Gain3/1
  Gain3/1 -> MATLAB Function3/6(ElectricalAngle)
  [M1_iqref] -> Delay/1
  [M1_idref] -> Delay1/1
  [M2_iqref] -> Delay2/1
  [M2_idref] -> Delay5/1
  Delay/1 -> MATLAB Function3/7(M1_iqref_prev)
  Delay1/1 -> MATLAB Function3/8(M1_idref_prev)
  Delay2/1 -> MATLAB Function3/9(M2_iqref_prev)
  Delay5/1 -> MATLAB Function3/10(M2_idref_prev)
  [Distributer_pulse] -> MATLAB Function3/17(pulse)
  Mean2/1 -> [Mean_loss]
  Bus Creator15/1 -> To Workspace6/1
  [Total_loss] -> Mean2/1
  [M1_loss] -> Bus Creator15/1  "M1_loss"
  [M2_loss] -> Bus Creator15/2  "M2_loss"
  [Total_loss] -> Bus Creator15/3  "Total_loss"
  [Mean_loss] -> Bus Creator15/4  "Mean_loss"
  Bus Creator16/1 -> To Workspace7/1
  [M1_iqref] -> Bus Creator16/1  "M1_iqref"
  [M1_idref] -> Bus Creator16/2  "M1_idref"
  [M2_iqref] -> Bus Creator16/3  "M2_iqref"
  [M2_idref] -> Bus Creator16/4  "M2_idref"
  From161/1 -> Scope16/4  "Mean_loss"
  From158/1 -> Scope16/3  "Total_loss"
  From160/1 -> Scope16/1  "M1_loss"
  From159/1 -> Scope16/2  "M2_loss"
  MATLAB Function3/9(M1_Iq_Opt_Proportional) -> [M1_Iq_opt_proportional]
  MATLAB Function3/10(M1_Id_Opt_Proportional) -> [M1_Id_opt_proportional]
  Gain14/1 -> Discrete-Time Integrator4/1
  Constant7/1 -> Sum15/2
  Discrete-Time Integrator4/State -> Sum15/1
  Saturation12/1 -> Compare To Zero2/1, MATLAB Function6/2(inputwave)
  Constant9/1 -> Gain14/1
  MATLAB Function6/1(outputwave) -> [Distributer]
  Compare To Zero2/1 -> MATLAB Function6/1(pulse)
  Sum15/1 -> Discrete-Time Integrator4/2
  Discrete-Time Integrator4/1 -> Saturation12/1
  Constant17/1 -> Switch6/1
  Constant27/1 -> Switch6/3
  Switch6/1 -> Edge Detector9/1
  [Distributer] -> Switch6/2
  From144/1 -> Bus Creator14/2  "M2_iqref"
  From171/1 -> Bus Creator19/1  "M1_ids"
  From170/1 -> Bus Creator20/2  "M2_idref"
  Bus Creator19/1 -> Scope19/1  "M1_ids"
  From172/1 -> Bus Creator20/1  "M2_ids"
  Bus Creator20/1 -> Scope19/2  "M2_ids"
  From146/1 -> Bus Creator13/1  "M1_iqs"
  From148/1 -> Bus Creator14/1  "M2_iqs"
  From131/1 -> Bus Creator19/2  "M1_idref"
  From143/1 -> Bus Creator13/2  "M1_iqref"
  Bus Creator14/1 -> Scope18/2  "M2_iqs"
  Bus Creator13/1 -> Scope18/1  "M1_iqs"
  Demux3/1 -> Mean Switching Frequency/4(In4)
  Demux3/5 -> Mean Switching Frequency/6(In6)
  Demux3/4 -> Terminator13/1
  Demux2/6 -> Terminator1/1
  Demux3/6 -> Terminator12/1
  Demux3/2 -> Terminator14/1
  Mean Switching Frequency/6(Out6) -> Display6/1
  Demux2/1 -> Mean Switching Frequency/1(In1)
  Mean Switching Frequency/3(Out3) -> Display3/1
  Demux2/5 -> Mean Switching Frequency/3(In3)
  Demux2/3 -> Mean Switching Frequency/2(In2)
  Demux2/4 -> Terminator10/1
  Demux2/2 -> Terminator11/1
  From6/1 -> Demux3/1
  Mean Switching Frequency/5(Out5) -> Display4/1
  Mean Switching Frequency/2(Out2) -> Display1/1
  Mean Switching Frequency/1(Out1) -> Display2/1
  From42/1 -> Demux2/1
  Mean Switching Frequency/4(Out4) -> Display5/1
  Demux3/3 -> Mean Switching Frequency/5(In5)
  Switch5/1 -> Edge Detector3/1
  [M1_wmech] -> Sample and Hold/1
  Edge Detector3/1 -> Sample and Hold/Trigger
  Constant37/1 -> Switch5/3
  Sawtooth Generator/1 -> Switch5/2
  Constant36/1 -> Switch5/1
  Sample and Hold/1 -> [wmech_lowrate]
  From165/1 -> Bus Creator18/2  "M2_opt"
  From166/1 -> Bus Creator17/1  "M1_iqref"
  From164/1 -> Bus Creator17/2  "M1_opt"
  Bus Creator17/1 -> Scope17/1
  Bus Creator18/1 -> Scope17/2
  From167/1 -> Bus Creator18/1  "M2_iqref"
  MATLAB Function4/3(Total_loss) -> [Total_cond_loss]  "total loss"
  MATLAB Function4/1(M1_loss) -> [M1_cond_loss]  "M1 loss"
  MATLAB Function4/2(M2_loss) -> [M2_cond_loss]  "M2 loss"
  Constant1/1 -> MATLAB Function4/7(Rs)
  [M1_Ia] -> MATLAB Function4/1(M1_ia)
  [M1_Ib] -> MATLAB Function4/2(M1_ib)
  [M1_Ic] -> MATLAB Function4/3(M1_ic)
  [M2_Ia] -> MATLAB Function4/4(M2_ia)
  [M2_Ib] -> MATLAB Function4/5(M2_ib)
  [M2_Ic] -> MATLAB Function4/6(M2_ic)
  [M1_wmech] -> Gain5/1
  Gain5/1 -> MATLAB Function3/15(ElectricalSpeed)
  Constant4/1 -> MATLAB Function3/16(FluxPM)
  Constant5/1 -> MATLAB Function3/5(Ls)
  MATLAB Function5/2(M2_magnetic_loss) -> [M2_core_loss]  "M2 loss"
  MATLAB Function5/1(M1_magnetic_loss) -> [M1_core_loss]  "M1 loss"
  MATLAB Function5/3(Total_loss) -> [Total_core_loss]  "total loss"
  [M1_wmech] -> Gain9/1
  Sum/1 -> [M1_loss]
  [M1_cond_loss] -> Sum/1
  [M1_core_loss] -> Sum/2
  [M2_cond_loss] -> Sum3/1
  Sum3/1 -> [M2_loss]
  [M2_core_loss] -> Sum3/2
  [Total_cond_loss] -> Sum7/1
  Sum7/1 -> [Total_loss]
  [Total_core_loss] -> Sum7/2
  From137/1 -> Scope3/1  "M1_cond_loss"
  From138/1 -> Scope3/2  "M1_core_loss"
  From140/1 -> Scope3/3  "M2_cond_loss"
  From139/1 -> Scope3/4  "M2_core_loss"
  From141/1 -> Scope3/5  "Total_cond_loss"
  From142/1 -> Scope3/6  "Total_core_loss"
  [M1_ids] -> MATLAB Function5/1(M1_ids)
  [M1_iqs] -> MATLAB Function5/2(M1_iqs)
  Constant26/1 -> MATLAB Function5/6(Ls)
  [M2_ids] -> MATLAB Function5/3(M2_ids)
  [M2_iqs] -> MATLAB Function5/4(M2_iqs)
  Constant6/1 -> MATLAB Function5/5(FluxPM)
  Gain9/1 -> MATLAB Function5/7(ElectricalSpeed)
  From156/1 -> Scope3/7  "Total_loss"
  [M1_cond_loss] -> Bus Creator15/5  "M1_cond_loss"
  [M1_core_loss] -> Bus Creator15/6  "M1_core_loss"
  [M2_cond_loss] -> Bus Creator15/7  "M2_cond_loss"
  [M2_core_loss] -> Bus Creator15/8  "M2_core_loss"
  [Total_cond_loss] -> Bus Creator15/9  "Total_cond_loss"
  [Total_core_loss] -> Bus Creator15/10  "Total_core_loss"
  MATLAB Function3/11(M2_Iq_Opt_Proportional) -> [M2_Iq_opt_proportional]
  MATLAB Function3/12(M2_Id_Opt_Proportional) -> [M2_Id_opt_proportional]
  [M1_Iq_opt_cost] -> MATLAB Function7/1(M1_Iq_opt_cost)
  [M1_Id_opt_cost] -> MATLAB Function7/2(M1_Id_opt_cost)
  [M2_Iq_opt_cost] -> MATLAB Function7/3(M2_Iq_opt_cost)
  [M2_Id_opt_cost] -> MATLAB Function7/4(M2_Id_opt_cost)
  [M1_Iq_opt_proportional] -> MATLAB Function7/5(M1_Iq_opt_proportional)
  [M1_Id_opt_proportional] -> MATLAB Function7/6(M1_Id_opt_proportional)
  [M2_Iq_opt_proportional] -> MATLAB Function7/7(M2_Iq_opt_proportional)
  [M2_Id_opt_proportional] -> MATLAB Function7/8(M2_Id_opt_proportional)
  Constant39/1 -> MATLAB Function7/10(M1_Id_opt_equal)
  [M1_Iq_opt_equal] -> MATLAB Function7/9(M1_Iq_opt_equal)
  [M2_Iq_opt_equal] -> MATLAB Function7/11(M2_Iq_opt_equal)
  Constant38/1 -> MATLAB Function7/12(M2_Id_opt_equal)
  Constant40/1 -> MATLAB Function7/13(selection)
  MATLAB Function7/1(M1_iqref) -> [M1_iqref]
  MATLAB Function7/2(M1_idref) -> [M1_idref]
  MATLAB Function7/3(M2_iqref) -> [M2_iqref]
  MATLAB Function7/4(M2_idref) -> [M2_idref]
  Ideal Switch/1 -> Terminator2/1
  [M1_Vca] -> Terminator3/1
  [M1_Vab] -> Terminator9/1
  [M1_Vbc] -> Terminator15/1
  [M2_Vab] -> Terminator16/1
  [M2_Vca] -> Terminator17/1
  [M2_Vbc] -> Terminator18/1
  [M1_vsq_actual] -> Terminator19/1
  [M1_vsd_actual] -> Terminator20/1
  [M2_vsq_actual] -> Terminator21/1
  [M2_vsd_actual] -> Terminator22/1
  [wref] -> Scope1/2  "wref"
  [M1_Iq_opt_proportional] -> Delay11/1
  [M1_Id_opt_proportional] -> Delay12/1
  [M2_Iq_opt_proportional] -> Delay13/1
  [M2_Id_opt_proportional] -> Delay14/1
  Delay11/1 -> MATLAB Function3/11(M1_Iq_Opt_Proportional_prev)
  Delay12/1 -> MATLAB Function3/12(M1_Id_Opt_Proportional_prev)
  Delay14/1 -> MATLAB Function3/14(M2_Id_Opt_Proportional_prev)
  Delay13/1 -> MATLAB Function3/13(M2_Iq_Opt_Proportional_prev)
  [M1_switching_pulse] -> Scope12/1  "M1_pulse"
  [M2_switching_pulse] -> Scope12/2  "M2_pulse"
  [M1_CarrierSignal] -> Scope13/1
  [M2_CarrierSignal] -> Scope13/2
  MATLAB Function8/2(counter) -> [counter_phase]
  [counter_phase] -> Delay16/1
  Delay16/1 -> MATLAB Function8/5(counter_prev)
  MATLAB Function8/1(phase) -> [phase], Scope15/1
  Clock8/1 -> Sample and Hold3/1
  [M2_switching_pulse] -> Sample and Hold3/Trigger
  Clock9/1 -> Sample and Hold4/1
  [M1_switching_pulse] -> Sample and Hold4/Trigger
  [phase] -> Delay17/1
  Delay17/1 -> MATLAB Function8/6(phase_prev)
  Sample and Hold4/1 -> [M1_int_moment], MATLAB Function8/3(time1)
  Sample and Hold3/1 -> [M2_int_moment], MATLAB Function8/4(time2)
  [M1_switching_pulse] -> MATLAB Function8/1(interrupt1)
  [M2_switching_pulse] -> MATLAB Function8/2(interrupt2)
  MATLAB Function2/1(outputwave) -> [M2_CarrierSignal]
  [wref] -> M1 Prediction/8(wref)
  M1 Prediction/13(Speed_Error) -> [M1_Speed_Error]
  M1 Prediction/14(Vds_Optimum) -> [M1_Vds_Optimum]
  M1 Prediction/15(Vqs_Optimum) -> [M1_Vqs_Optimum]
  [M1_Speed_Error] -> Delay23/1
  Delay23/1 -> M1 Prediction/21(Speed_Error_prev)
  [M1_Vds_Optimum] -> Delay25/1
  [M1_Vqs_Optimum] -> Delay24/1
  Delay24/1 -> M1 Prediction/23(Vqs_Optimum_prev)
  Delay25/1 -> M1 Prediction/22(Vds_Optimum_prev)
  [wref] -> M2 Prediction/8(wref)
  M2 Prediction/3(DutyC) -> [M2_DutyC]
  M2 Prediction/7(Vds_Optimum) -> [M2_Vds_Optimum]
  M2 Prediction/8(Vqs_Optimum) -> [M2_Vqs_Optimum]
  M2 Prediction/6(Speed_Error) -> [M2_Speed_Error]
  Delay26/1 -> M2 Prediction/23(Vds_Optimum_prev)
  Delay21/1 -> M2 Prediction/22(Speed_Error_prev)
  Delay27/1 -> M2 Prediction/24(Vqs_Optimum_prev)
  [M2_Speed_Error] -> Delay21/1
  [M2_Vds_Optimum] -> Delay26/1
  [M2_Vqs_Optimum] -> Delay27/1
  Constant45/1 -> MATLAB Function9/4(Ki)
  Discrete-Time Integrator1/State -> Sum11/1
  Constant48/1 -> MATLAB Function9/7(Sat)
  [wref] -> MATLAB Function9/2(Ref)
  Delay28/1 -> MATLAB Function9/9(OutputPrev)
  [PI_IQ_INTERRUPT] -> MATLAB Function9/1(InterruptSignal)
  [PI_error] -> Delay29/1
  Delay29/1 -> MATLAB Function9/8(ErrorPrev)
  MATLAB Function9/2(Error) -> [PI_error]
  [PI_output] -> Delay28/1
  Switch7/1 -> Edge Detector6/1
  MATLAB Function9/1(Output) -> [PI_output]
  [PI_IQ_SIGNAL] -> Switch7/2
  Constant41/1 -> Sum11/2
  Constant47/1 -> MATLAB Function9/6(Ts)
  Constant43/1 -> Switch7/1
  [wmech_lowrate] -> MATLAB Function9/3(Measured)
  Edge Detector6/1 -> [PI_IQ_INTERRUPT]
  Gain12/1 -> Discrete-Time Integrator1/1
  Constant44/1 -> Switch7/3
  Sum11/1 -> Discrete-Time Integrator1/2
  MATLAB Function10/1(outputwave) -> [PI_IQ_SIGNAL]
  Discrete-Time Integrator1/1 -> Saturation3/1
  Constant42/1 -> Gain12/1
  Constant46/1 -> MATLAB Function9/5(Kp)
  Saturation3/1 -> Compare To Zero3/1, MATLAB Function10/2(inputwave)
  Compare To Zero3/1 -> MATLAB Function10/1(pulse)
  Switch8/1 -> Edge Detector5/1
  Edge Detector5/1 -> [M1_switching_pulse], [M1_sampling_pulse]
  Constant50/1 -> Switch8/3
  [M1_CarrierSignal] -> Switch8/2
  Constant49/1 -> Switch8/1
  Constant51/1 -> Switch9/1
  [M2_CarrierSignal] -> Switch9/2
  Constant52/1 -> Switch9/3
  Edge Detector1/1 -> [M2_switching_pulse], [M2_sampling_pulse]
  Switch9/1 -> Edge Detector1/1
  [M2_Ib] -> Sample and Hold11/1
  [M1_sampling_pulse] -> Sample and Hold9/Trigger, Sample and Hold12/Trigger, Sample and Hold13/Trigger
  Sample and Hold10/1 -> module 2 abc to dq1/3(ics)
  Sample and Hold12/1 -> module 1 abc to dq1/2(ibs)
  [M2_Ia] -> Sample and Hold14/1
  Sample and Hold13/1 -> module 1 abc to dq1/1(ias)
  [M1_Ic] -> Sample and Hold9/1
  [M2_sampling_pulse] -> Sample and Hold10/Trigger, Sample and Hold11/Trigger, Sample and Hold14/Trigger
  module 2 abc to dq1/3(i0) -> Terminator24/1
  [M1_Ia] -> Sample and Hold13/1
  Sample and Hold11/1 -> module 2 abc to dq1/2(ibs)
  [M1_thetam] -> Gain13/1
  Gain15/1 -> module 2 abc to dq1/4(ref_frame_position)
  [M2_thetam] -> Gain15/1
  module 1 abc to dq1/3(i0) -> Terminator23/1
  Sample and Hold14/1 -> module 2 abc to dq1/1(ias)
  module 2 abc to dq1/2(iqs) -> [M2_iqs]
  module 1 abc to dq1/1(ids) -> [M1_ids]
  module 2 abc to dq1/1(ids) -> [M2_ids]
  Sample and Hold9/1 -> module 1 abc to dq1/3(ics)
  [M2_Ic] -> Sample and Hold10/1
  module 1 abc to dq1/2(iqs) -> [M1_iqs]
  Gain13/1 -> module 1 abc to dq1/4(ref_frame_position)
  [M1_Ib] -> Sample and Hold12/1
  [M1_fsw_out] -> M2 Prediction/26(M1_fsw)
  [M2_fsw_out] -> Delay6/1
  [phase] -> M2 Prediction/25(fsw_phase)
  Delay6/1 -> M2 Prediction/27(M2_fsw_prev)
  [M1_int_moment] -> M2 Prediction/28(M1_int_moment)
  [M2_int_moment] -> M2 Prediction/29(M2_int_moment)
  Switch4/1 -> Edge Detector8/1
  Edge Detector8/1 -> Terminator/1
  Switch2/1 -> Edge Detector7/1
  Edge Detector7/1 -> Terminator8/1
  Edge Detector9/1 -> [Distributer_pulse]
  Sum13/1 -> [M2_Iq_opt_equal]
  Gain11/1 -> [M1_Iq_opt_equal]
  [M1_iqs] -> Sum13/2
  [PI_output] -> Sum13/1, Gain11/1
  MATLAB Function/1(a) -> Scope14/1
  MATLAB Function/2(b) -> Scope14/2
  MATLAB Function/3(c) -> Scope14/3
  From49/1 -> MATLAB Function/1(d)
  From94/1 -> MATLAB Function/2(q)
  Constant53/1 -> MATLAB Function/3(zero)
  From122/1 -> Gain2/1
  Gain2/1 -> MATLAB Function/4(angle)
  Switch11/1 -> MATLAB Function3/1(iqref)
  Sample and Hold1/1 -> [M1_magneticloss]
  MATLAB Function3/3(M1_magneticloss) -> Sample and Hold1/1
  MATLAB Function3/4(M2_magneticloss) -> Sample and Hold2/1
  Sample and Hold2/1 -> [M2_magneticloss]
  [Distributer_pulse] -> Sample and Hold5/Trigger, Sample and Hold6/Trigger, Sample and Hold1/Trigger, Sample and Hold2/Trigger
  Sample and Hold5/1 -> [M1_copper_loss]
  Sample and Hold6/1 -> [M2_copper_loss]
  MATLAB Function3/2(M2_copperloss) -> Sample and Hold6/1
  MATLAB Function3/1(M1_copperloss) -> Sample and Hold5/1
  From245/1 -> Scope24/1  "M1_iqs"
  From244/1 -> Scope25/1  "M1_ids"
  From242/1 -> Scope24/2  "M1_iq_reference"
  From243/1 -> Scope25/2  "M1_id_reference"
  From247/1 -> Scope26/1  "M2_iqs"
  From246/1 -> Scope27/1  "M2_ids"
  From241/1 -> Scope26/2  "M2_iq_reference"
  From240/1 -> Scope27/2  "M2_id_reference"
  Current Measurement7/1 -> [Idc_meas]
  Product/1 -> Scope23/1
  [M2_copper_loss] -> Scope22/2
  From239/1 -> Product/1
  From235/1 -> Scope21/2
  [M1_copper_loss] -> Scope22/1
  From234/1 -> Scope21/1
  From238/1 -> Product/2
  [PI_output] -> Scope20/3
  From248/1 -> MATLAB Function11/1(M1_id)
  From249/1 -> MATLAB Function11/2(M1_iq)
  From250/1 -> MATLAB Function11/3(M2_id)
  From251/1 -> MATLAB Function11/4(M2_iq)
  MATLAB Function11/1(M1_Torque) -> Mux/1  "M1_Torque_Calculated"
  MATLAB Function11/2(M2_Torque) -> Mux2/1  "M2_Torque_Calculated"
  From252/1 -> Mux/2  "M1_Torque_Measured"
  From253/1 -> Mux2/2  "M2_Torque_Measured"
  Mux2/1 -> Scope28/2
  Mux/1 -> Scope28/1
  MATLAB Function3/13(weight) -> Scope29/1
  Constant54/1 -> Scope20/4
  MATLAB Function3/14(M1_lossfactor) -> [M1_lossfactor]
  MATLAB Function3/15(M2_lossfactor) -> [M2_lossfactor]
  [M1_lossfactor] -> Delay22/1
  [M2_lossfactor] -> Delay30/1
  Delay22/1 -> MATLAB Function3/18(M1_lossfactor_prev)
  Delay30/1 -> MATLAB Function3/19(M2_lossfactor_prev)
  [M1_lossfactor] -> Scope30/1
  [M2_lossfactor] -> Scope30/2
  [M1_copper_loss] -> Mean4/1, Sum14/1
  [M2_copper_loss] -> Sum14/2, Mean1/1
  Sum14/1 -> Mean3/1
  Mean1/1 -> Scope31/2  "M2_loss"
  Mean4/1 -> Scope31/1  "M1_loss"
  Mean3/1 -> Scope31/3  "Total loss"
  From261/1 -> MATLAB Function12/2(M1_iq)  "M1_iqs"
  From260/1 -> MATLAB Function12/1(M1_id)  "M1_ids"
  From263/1 -> MATLAB Function12/4(M2_iq)  "M2_iqs"
  From262/1 -> MATLAB Function12/3(M2_id)  "M2_ids"
  Mean6/1 -> Scope32/3  "Total loss"
  Mean5/1 -> Scope32/2  "M2_loss"
  Sum16/1 -> Scope33/3, Mean6/1
  Mean7/1 -> Scope32/1  "M1_loss"
  MATLAB Function12/2(M2_copper_loss) -> Scope33/2, Mean5/1, Sum16/2
  MATLAB Function12/1(M1_copper_loss) -> Scope33/1, Mean7/1, Sum16/1
  M2 Prediction/9(FswPhases) -> Sample and Hold7/1
  Sample and Hold7/1 -> Scope34/1
  [M2_switching_pulse] -> Sample and Hold19/Trigger, Sample and Hold20/Trigger, Sample and Hold24/Trigger, Sample and Hold23/Trigger, Sample and Hold22/Trigger, Sample and Hold21/Trigger, Sample and Hold7/Trigger
  M1 Prediction/5(p5_out) -> Sample and Hold8/1
  M1 Prediction/4(p4_out) -> Sample and Hold15/1
  M1 Prediction/3(p3_out) -> Sample and Hold16/1
  M1 Prediction/2(p2_out) -> Sample and Hold17/1
  M1 Prediction/1(p1_out) -> Sample and Hold18/1
  [M1_switching_pulse] -> Sample and Hold16/Trigger, Sample and Hold29/Trigger, Sample and Hold28/Trigger, Sample and Hold8/Trigger, Sample and Hold15/Trigger, Sample and Hold17/Trigger, Sample and Hold18/Trigger
  M2 Prediction/10(p1_out) -> Sample and Hold19/1
  M2 Prediction/11(p2_out) -> Sample and Hold20/1
  M2 Prediction/12(p3_out) -> Sample and Hold21/1
  M2 Prediction/13(p4_out) -> Sample and Hold22/1
  M2 Prediction/15(p6_out) -> Sample and Hold24/1
  M2 Prediction/14(p5_out) -> Sample and Hold23/1
  [wmech_lowrate] -> Delay31/1
  Delay31/1 -> M2 Prediction/10(ShaftAngularSpeed_prev)
  M2 Prediction/16(filter_out) -> [M1_filter_out]
  [M1_filter_out] -> Delay32/1
  Delay32/1 -> M2 Prediction/30(filter_out_prev)
  [M2_filter_out] -> Delay33/1
  Delay33/1 -> M1 Prediction/24(filter_out_prev)
  M1 Prediction/16(filter_out) -> [M2_filter_out]
  Multimeter/1 -> MATLAB Function13/1(Switch_Current)
  [M1_fsw_out] -> MATLAB Function13/2(fsw)
  MATLAB Function13/1(ConductionLoss) -> [M1_ConductionLoss], Scope37/1
  MATLAB Function13/2(SwitchingLoss) -> [M1_FswLoss], Scope37/2
  MATLAB Function14/2(SwitchingLoss) -> [M2_FswLoss], Scope38/2
  Multimeter1/1 -> MATLAB Function14/1(Switch_Current)
  [M2_fsw_out] -> MATLAB Function14/2(fsw)
  MATLAB Function14/1(ConductionLoss) -> [M2_ConductionLoss], Scope38/1
  [M2_ConductionLoss] -> Bus Creator21/3  "M2Cond"
  [M2_FswLoss] -> Bus Creator21/4  "M2Fsw"
  [M1_FswLoss] -> Bus Creator21/2  "M1Fsw"
  [M1_ConductionLoss] -> Bus Creator21/1  "M1Cond"
  Bus Creator21/1 -> To Workspace8/1
  Sample and Hold26/1 -> MATLAB Function15/2(moment2)
  Sample and Hold25/1 -> MATLAB Function15/1(moment1)
  Clock6/1 -> Sample and Hold26/1, Sample and Hold25/1
  [M1_switching_pulse] -> Sample and Hold25/Trigger
  [M2_switching_pulse] -> Sample and Hold27/Trigger, Sample and Hold26/Trigger
  MATLAB Function15/1(phase) -> [fsw_phases], Scope39/1
  [M1_fsw_out] -> Sample and Hold27/1
  Sample and Hold27/1 -> MATLAB Function15/3(fsw1)
  [fsw_phases] -> Bus Creator22/1  "fsw_phases"
  Bus Creator22/1 -> To Workspace/1
  Sample and Hold19/1 -> [M2_P1_out]  "p1"
  Sample and Hold20/1 -> [M2_P2_out]  "p2"
  Sample and Hold21/1 -> [M2_P3_out]  "p3"
  Sample and Hold22/1 -> [M2_P4_out]  "p4"
  Sample and Hold23/1 -> [M2_P5_out]  "p5"
  Sample and Hold24/1 -> [M2_P6_out]  "p6"
  [M2_P1_out] -> Scope36/1
  [M2_P2_out] -> Scope36/2
  [M2_P3_out] -> Scope36/3
  [M2_P4_out] -> Scope36/4
  [M2_P5_out] -> Scope36/5
  [M2_P6_out] -> Scope36/6
  Sample and Hold18/1 -> [M1_P1_out]  "p1"
  Sample and Hold17/1 -> [M1_P2_out]  "p2"
  Sample and Hold16/1 -> [M1_P3_out]  "p3"
  Sample and Hold15/1 -> [M1_P4_out]  "p4"
  Sample and Hold8/1 -> [M1_P5_out]  "p5"
  [M1_P5_out] -> Bus Creator22/6  "M1_P5_out"
  [M1_P4_out] -> Bus Creator22/5  "M1_P4_out"
  [M1_P3_out] -> Bus Creator22/4  "M1_P3_out"
  [M1_P2_out] -> Bus Creator22/3  "M1_P2_out"
  [M1_P1_out] -> Bus Creator22/2  "M1_P1_out"
  [M2_P6_out] -> Bus Creator22/12  "M2_P6_out"
  [M2_P5_out] -> Bus Creator22/11  "M2_P5_out"
  [M2_P4_out] -> Bus Creator22/10  "M2_P4_out"
  [M2_P2_out] -> Bus Creator22/8  "M2_P2_out"
  [M2_P1_out] -> Bus Creator22/7  "M2_P1_out"
  [M2_P3_out] -> Bus Creator22/9  "M2_P3_out"
  [M1_idref] -> Scope35/2
  [M1_ids] -> Scope35/1  "M1_ids"
  [M1_P1_out] -> Scope40/1  "M1_P1_out"
  [M1_P2_out] -> Scope40/2  "M1_P2_out"
  [M1_P3_out] -> Scope40/3  "M1_P3_out"
  [M1_P4_out] -> Scope40/4  "M1_P4_out"
  [M1_P5_out] -> Scope40/5  "M1_P5_out"
  [M1_wmech] -> Mechanical Subsystem/1(In1)
  Constant56/1 -> Switch11/3
  Constant55/1 -> Switch11/1
  Clock7/1 -> Switch11/2
  M1 Prediction/6(iq_2_out) -> Sample and Hold28/1
  Sample and Hold28/1 -> [iq_2_out]  "p5"
  [iq_2_out] -> Scope40/6
  M1 Prediction/7(iq_2_store) -> Sample and Hold29/1
  Sample and Hold29/1 -> [iq_2_store]  "p5"
  From309/1 -> Demux/1
  Demux/2 -> Scope42/2  "2"
  Demux/8 -> Scope42/8  "8"
  Demux/1 -> Scope42/1  "1"
  Demux/5 -> Scope42/5  "5"
  Demux/10 -> Scope42/10  "10"
  Demux/3 -> Scope42/3  "3"
  Demux/4 -> Scope42/4  "4"
  Demux/6 -> Scope42/6  "6"
  Demux/9 -> Scope42/9  "9"
  Demux/7 -> Scope42/7  "7"
  Demux1/7 -> Error/7  "7"
  Demux1/9 -> Error/9  "9"
  Demux1/5 -> Error/5  "5"
  Demux1/4 -> Error/4  "4"
  Demux1/1 -> Error/1  "1"
  Demux1/6 -> Error/6  "6"
  Demux1/3 -> Error/3  "3"
  Demux1/10 -> Error/10  "10"
  Demux1/8 -> Error/8  "8"
  Demux1/2 -> Error/2  "2"
  From311/1 -> Sum18/1  "M1_iqref"
  From310/1 -> Sum18/2
  Sum18/1 -> Demux1/1
  connections:
  DCLINK_Cap/LConn1 -- Current Measurement/LConn1 -- Voltage Measurement3/LConn1
  Controlled Voltage Source/RConn1 -- Rin/RConn1
  Current Measurement3/RConn1 -- Permanent Magnet Synchronous Machine/LConn4
  Permanent Magnet Synchronous Machine/LConn3 -- Current Measurement2/RConn1
  Permanent Magnet Synchronous Machine/LConn2 -- Current Measurement1/RConn1
  Current Measurement1/LConn1 -- Ideal Switch/RConn1 -- Series RLC Branch/RConn1
  Mechanical Subsystem/LConn1 -- Permanent Magnet Synchronous Machine/LConn1 -- Permanent Magnet Synchronous Machine1/LConn1
  Permanent Magnet Synchronous Machine1/LConn4 -- Current Measurement6/RConn1
  Current Measurement6/LConn1 -- Inverter2/LConn3 -- Voltage Measurement5/LConn2 -- Voltage Measurement6/LConn1
  Permanent Magnet Synchronous Machine1/LConn3 -- Current Measurement5/RConn1
  Current Measurement2/LConn1 -- Voltage Measurement1/LConn1 -- Voltage Measurement/LConn2 -- Inverter1/LConn2
  Current Measurement4/RConn1 -- Permanent Magnet Synchronous Machine1/LConn2
  Current Measurement/RConn1 -- Current Measurement7/LConn1 -- Rin/LConn1
  Voltage Measurement2/LConn2 -- Ideal Switch/LConn1 -- Series RLC Branch/LConn1 -- Voltage Measurement/LConn1 -- Inverter1/LConn1
  DCLINK_Cap/RConn1 -- Controlled Voltage Source/LConn1 -- Voltage Measurement3/LConn2 -- Inverter2/RConn2 -- Inverter1/RConn2
  Current Measurement4/LConn1 -- Inverter2/LConn1 -- Voltage Measurement4/LConn1 -- Voltage Measurement6/LConn2
  Current Measurement5/LConn1 -- Inverter2/LConn2 -- Voltage Measurement5/LConn1 -- Voltage Measurement4/LConn2
  Voltage Measurement1/LConn2 -- Inverter1/LConn3 -- Voltage Measurement2/LConn1 -- Current Measurement3/LConn1
  Inverter2/RConn1 -- Current Measurement7/RConn1 -- Inverter1/RConn1
